simulink model "v1bate3"  (Simulink 8.8)
settings: Solver=ode3  StartTime=0.0  StopTime=inf  FixedStep=0.001  RelTol=1e-3  EnableMultiTasking=on
undefined symbols (not defined in the file): mdaadlink6208
libraries: simulink x19
(part 2 of 2)

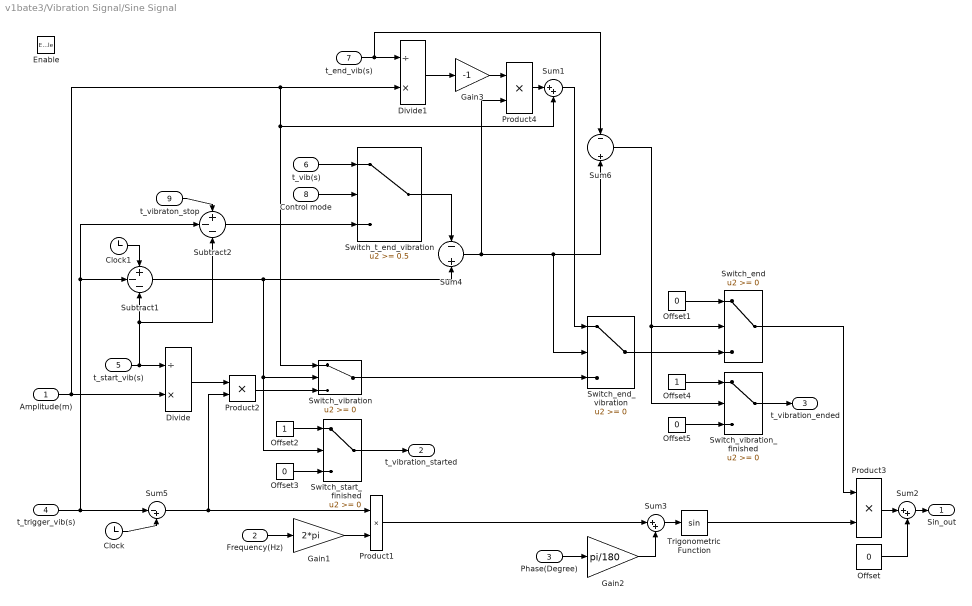
== system v1bate3/Vibration Signal/Sine Signal ==
  Amplitude(m) : Inport
  Frequency(Hz) : Inport  Port=2
  Phase(Degree) : Inport  Port=3
  t_trigger_vib(s) : Inport  Port=4
  t_start_vib(s) : Inport  Port=5
  t_vib(s) : Inport  Port=6
  t_end_vib(s) : Inport  Port=7
  Control mode : Inport  Port=8
  t_vibraton_stop : Inport  Port=9
  Enable : EnablePort  StatesWhenEnabling=reset
  Clock : Clock
      settings: Decimation=100
  Clock1 : Clock
      settings: Decimation=100
  Divide : Product  Inputs=/*
  Divide1 : Product  Inputs=/*
  Gain1 : Gain  Gain=2*pi  SaturateOnIntegerOverflow=on  OutDataTypeStr=Inherit: Same as input  ParamDataTypeStr=Inherit: Same as input
  Gain2 : Gain  Gain=pi/180  SaturateOnIntegerOverflow=on  OutDataTypeStr=Inherit: Same as input  ParamDataTypeStr=Inherit: Same as input
  Gain3 : Gain  Gain=-1  SaturateOnIntegerOverflow=on  OutDataTypeStr=Inherit: Same as input  ParamDataTypeStr=Inherit: Same as input
  Offset{,1,3,5} (4 alike) : Constant  Value=0
  Offset2 : Constant
  Offset4 : Constant
  Product1 : Product  SaturateOnIntegerOverflow=on  OutDataTypeStr=Inherit: Same as first input
  Product2 : Product  RndMeth=Zero
  Product3 : Product  SaturateOnIntegerOverflow=on  OutDataTypeStr=Inherit: Same as first input
  Product4 : Product  RndMeth=Zero
  Subtract1 : Sum  Inputs=+--
  Subtract2 : Sum  Inputs=+--
  Sum1 : Sum  Inputs=|++  SaturateOnIntegerOverflow=on
  Sum2 : Sum  Inputs=|++  SaturateOnIntegerOverflow=on
  Sum3 : Sum  Inputs=|++  SaturateOnIntegerOverflow=on
  Sum4 : Sum  Inputs=-+  SaturateOnIntegerOverflow=on
  Sum5 : Sum  Inputs=|-+  SaturateOnIntegerOverflow=on
  Sum6 : Sum  Inputs=-||+  SaturateOnIntegerOverflow=on
  Switch_end : Switch
  Switch_end_vibration : Switch
  Switch_start_finished : Switch
  Switch_t_end_vibration : Switch  Threshold=0.5
  Switch_vibration : Switch
  Switch_vibration_finished : Switch
  Trigonometric Function : Trigonometry
  Sin_out : Outport
  t_vibration_started : Outport  Port=2
  t_vibration_ended : Outport  Port=3
  wires:
  Product3/1 -> Sum2/1
  Sum2/1 -> Sin_out/1
  Offset/1 -> Sum2/2
  Frequency(Hz)/1 -> Gain1/1
  Sum3/1 -> Trigonometric Function/1
  Trigonometric Function/1 -> Product3/2
  Product1/1 -> Sum3/1
  Gain2/1 -> Sum3/2
  Phase(Degree)/1 -> Gain2/1
  t_trigger_vib(s)/1 -> Sum5/1, Subtract2/2, Subtract1/2
  Sum5/1 -> Product1/1, Product2/2
  Gain1/1 -> Product1/2
  Clock1/1 -> Subtract1/1
  Subtract1/1 -> Sum4/2, Switch_start_finished/2, Switch_vibration/2
  Product2/1 -> Switch_vibration/3
  Switch_vibration/1 -> Switch_end_vibration/3
  Switch_end_vibration/1 -> Switch_end/3
  Switch_end/1 -> Product3/1
  Sum6/1 -> Switch_vibration_finished/2, Switch_end/2
  Divide1/1 -> Gain3/1
  Gain3/1 -> Product4/1
  Offset1/1 -> Switch_end/1
  Sum4/1 -> Product4/2, Switch_end_vibration/2, Sum6/2
  t_end_vib(s)/1 -> Divide1/1, Sum6/1
  Product4/1 -> Sum1/1
  Divide/1 -> Product2/1
  t_start_vib(s)/1 -> Divide/1, Subtract1/3, Subtract2/3
  Amplitude(m)/1 -> Divide/2, Divide1/2, Switch_vibration/1, Sum1/2
  Sum1/1 -> Switch_end_vibration/1
  Switch_start_finished/1 -> t_vibration_started/1
  Offset2/1 -> Switch_start_finished/1
  Offset3/1 -> Switch_start_finished/3
  Switch_vibration_finished/1 -> t_vibration_ended/1
  Offset4/1 -> Switch_vibration_finished/1
  Offset5/1 -> Switch_vibration_finished/3
  Clock/1 -> Sum5/2
  Control mode/1 -> Switch_t_end_vibration/2
  t_vib(s)/1 -> Switch_t_end_vibration/1
  t_vibraton_stop/1 -> Subtract2/1
  Subtract2/1 -> Switch_t_end_vibration/3
  Switch_t_end_vibration/1 -> Sum4/1

== system v1bate3/Vibration Signal/Vibration start trigger ==
  In1 : Inport
  Trigger : TriggerPort  VariantControl=Variant
  Out1 : Outport
  wires:
  In1/1 -> Out1/1

== system v1bate3/Vibration Signal/Vibration stop trigger ==
  In1 : Inport
  Trigger : TriggerPort  VariantControl=Variant
  Out1 : Outport
  wires:
  In1/1 -> Out1/1

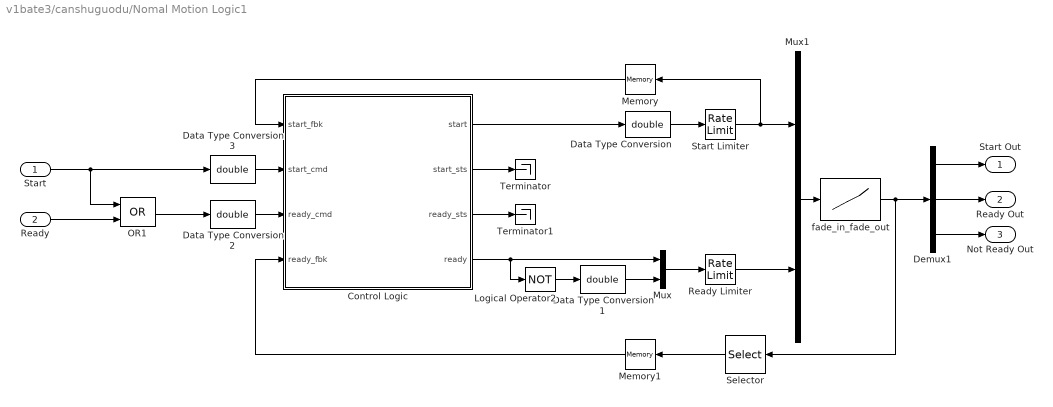
== system v1bate3/canshuguodu/Nomal Motion Logic1 ==
  Start : Inport
  Ready : Inport  Port=2
  Control Logic : Stateflow chart  TreatAsAtomicUnit=on
  Data Type Conversion{,1..3} (4 alike) : DataTypeConversion  OutDataTypeStr=double  SaturateOnIntegerOverflow=on  RndMeth=Zero
  Demux1 : Demux  Outputs=3
  Logical Operator2 : Logic  Operator=NOT  Inputs=3  AllPortsSameDT=off
  Memory : Memory
  Memory1 : Memory
  Mux : Mux  Inputs=2
  Mux1 : Mux  Inputs=2
  OR1 : Logic  Operator=OR  AllPortsSameDT=off
  Ready Limiter : RateLimiter  RisingSlewLimit=1/20  FallingSlewLimit=-1/20
  Selector : Selector  InputPortWidth=3  IndexOptions=Index vector (dialog)  Indices=[2]  OutputSizes=1
  Start Limiter : RateLimiter  RisingSlewLimit=1/3  FallingSlewLimit=-1/3
  Terminator : Terminator
  Terminator1 : Terminator
  fade_in_fade_out : Lookup  InputValues=[0:0.001:1]  Table=(sin(([0:0.001:1]*2-1)*pi/2)+1)/2  SaturateOnIntegerOverflow=on
  Start Out : Outport
  Ready Out : Outport  Port=2
  Not Ready Out : Outport  Port=3
  wires:
  Ready/1 -> OR1/2
  Start/1 -> OR1/1, Data Type Conversion3/1
  Control Logic/3(ready_sts) -> Terminator1/1
  Control Logic/2(start_sts) -> Terminator/1
  OR1/1 -> Data Type Conversion2/1
  Data Type Conversion3/1 -> Control Logic/2(start_cmd)
  Demux1/3 -> Not Ready Out/1
  Demux1/1 -> Start Out/1
  Demux1/2 -> Ready Out/1
  Data Type Conversion/1 -> Start Limiter/1
  Start Limiter/1 -> Mux1/1, Memory/1
  Control Logic/1(start) -> Data Type Conversion/1
  Control Logic/4(ready) -> Logical Operator2/1, Mux/1
  Logical Operator2/1 -> Data Type Conversion1/1
  Mux/1 -> Ready Limiter/1
  Ready Limiter/1 -> Mux1/2
  Mux1/1 -> fade_in_fade_out/1
  fade_in_fade_out/1 -> Selector/1, Demux1/1
  Memory/1 -> Control Logic/1(start_fbk)
  Memory1/1 -> Control Logic/4(ready_fbk)
  Data Type Conversion1/1 -> Mux/2
  Data Type Conversion2/1 -> Control Logic/3(ready_cmd)
  Selector/1 -> Memory1/1

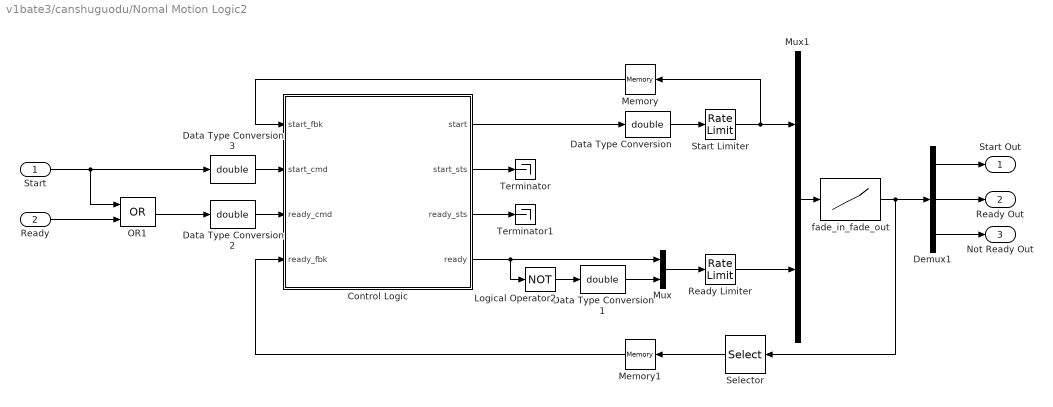
== system v1bate3/canshuguodu/Nomal Motion Logic2 ==
  Start : Inport
  Ready : Inport  Port=2
  Control Logic : Stateflow chart  TreatAsAtomicUnit=on
  Data Type Conversion{,1..3} (4 alike) : DataTypeConversion  OutDataTypeStr=double  SaturateOnIntegerOverflow=on  RndMeth=Zero
  Demux1 : Demux  Outputs=3
  Logical Operator2 : Logic  Operator=NOT  Inputs=3  AllPortsSameDT=off
  Memory : Memory
  Memory1 : Memory
  Mux : Mux  Inputs=2
  Mux1 : Mux  Inputs=2
  OR1 : Logic  Operator=OR  AllPortsSameDT=off
  Ready Limiter : RateLimiter  RisingSlewLimit=1/20  FallingSlewLimit=-1/20
  Selector : Selector  InputPortWidth=3  IndexOptions=Index vector (dialog)  Indices=[2]  OutputSizes=1
  Start Limiter : RateLimiter  RisingSlewLimit=1/3  FallingSlewLimit=-1/3
  Terminator : Terminator
  Terminator1 : Terminator
  fade_in_fade_out : Lookup  InputValues=[0:0.001:1]  Table=(sin(([0:0.001:1]*2-1)*pi/2)+1)/2  SaturateOnIntegerOverflow=on
  Start Out : Outport
  Ready Out : Outport  Port=2
  Not Ready Out : Outport  Port=3
  wires:
  Ready/1 -> OR1/2
  Start/1 -> OR1/1, Data Type Conversion3/1
  Control Logic/3(ready_sts) -> Terminator1/1
  Control Logic/2(start_sts) -> Terminator/1
  OR1/1 -> Data Type Conversion2/1
  Data Type Conversion3/1 -> Control Logic/2(start_cmd)
  Demux1/3 -> Not Ready Out/1
  Demux1/1 -> Start Out/1
  Demux1/2 -> Ready Out/1
  Data Type Conversion/1 -> Start Limiter/1
  Start Limiter/1 -> Mux1/1, Memory/1
  Control Logic/1(start) -> Data Type Conversion/1
  Control Logic/4(ready) -> Logical Operator2/1, Mux/1
  Logical Operator2/1 -> Data Type Conversion1/1
  Mux/1 -> Ready Limiter/1
  Ready Limiter/1 -> Mux1/2
  Mux1/1 -> fade_in_fade_out/1
  fade_in_fade_out/1 -> Selector/1, Demux1/1
  Memory/1 -> Control Logic/1(start_fbk)
  Memory1/1 -> Control Logic/4(ready_fbk)
  Data Type Conversion1/1 -> Mux/2
  Data Type Conversion2/1 -> Control Logic/3(ready_cmd)
  Selector/1 -> Memory1/1

== system v1bate3/huituixinhao1/Triggered Subsystem2 ==
  Trigger : TriggerPort  VariantControl=Variant
  Digital Clock : DigitalClock  SampleTime=-1
  force-single1 : Outport
  wires:
  Digital Clock/1 -> force-single1/1

== system v1bate3/jiechuhuitui2/Triggered Subsystem1 ==
  Trigger : TriggerPort  VariantControl=Variant
  c3 : Constant
  force-single1 : Outport
  wires:
  c3/1 -> force-single1/1

== system v1bate3/jiechuhuitui2/Triggered Subsystem2 ==
  Trigger : TriggerPort  TriggerType=falling  VariantControl=Variant
  c3 : Constant
  force-single1 : Outport
  wires:
  c3/1 -> force-single1/1

== system v1bate3/single with d/Triggered Subsystem1 ==
  Trigger : TriggerPort  VariantControl=Variant
  c7 : Constant
  tingzhenxinhao : Outport
  wires:
  c7/1 -> tingzhenxinhao/1

== system v1bate3/single with d/Triggered Subsystem2 ==
  Trigger : TriggerPort  VariantControl=Variant
  Digital Clock : DigitalClock  SampleTime=-1
  force-single1 : Outport
  wires:
  Digital Clock/1 -> force-single1/1

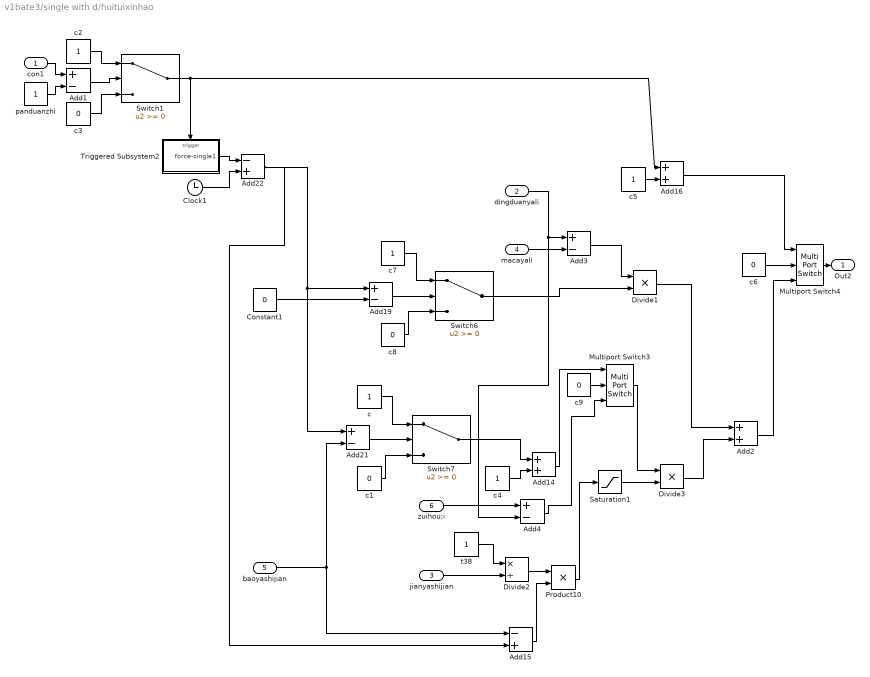
== system v1bate3/single with d/huituixinhao ==
  con1 : Inport
  dingduanyali : Inport  Port=2
  jianyashijian : Inport  Port=3
  macayali : Inport  Port=4
  baoyashijian : Inport  Port=5
  zuihou;i : Inport  Port=6
  Add{1,3..4,19,21} (5 alike) : Sum  Inputs=+-
  Add14 : Sum
  Add15 : Sum  Inputs=-+
  Add16 : Sum
  Add2 : Sum
  Add22 : Sum  Inputs=-+
  Clock1 : Clock
  Constant1 : Constant  Value=0
  Divide1 : Product  Inputs=**
  Divide2 : Product  Inputs=*/
  Divide3 : Product  Inputs=**
  Multiport Switch3 : MultiPortSwitch  Inputs=2
  Multiport Switch4 : MultiPortSwitch  Inputs=2
  Product10 : Product  RndMeth=Zero
  Saturation1 : Saturate  UpperLimit=1  LowerLimit=-1
  Switch1 : Switch
  Switch6 : Switch
  Switch7 : Switch
  Triggered Subsystem2 : Subsystem  TreatAsAtomicUnit=on
  c{,2,4..5,7} (5 alike) : Constant
  c{1,3,6,8..9} (5 alike) : Constant  Value=0
  panduanzhi : Constant
  t38 : Constant
  Out2 : Outport
  wires:
  Triggered Subsystem2/1(force-single1) -> Add22/1
  Clock1/1 -> Add22/2
  t38/1 -> Divide2/1
  Product10/1 -> Saturation1/1
  Saturation1/1 -> Divide3/2
  Divide2/1 -> Product10/1
  Add15/1 -> Product10/2
  baoyashijian/1 -> Add15/1, Add21/2
  Multiport Switch3/1 -> Divide3/1
  c/1 -> Switch7/1
  c1/1 -> Switch7/3
  Add21/1 -> Switch7/2
  c9/1 -> Multiport Switch3/2
  Add14/1 -> Multiport Switch3/1
  Switch7/1 -> Add14/1
  c4/1 -> Add14/2
  Add22/1 -> Add15/2, Add21/1, Add19/1
  panduanzhi/1 -> Add1/2
  Add1/1 -> Switch1/2
  c2/1 -> Switch1/1
  c3/1 -> Switch1/3
  Switch1/1 -> Triggered Subsystem2/Trigger, Add16/1
  Add4/1 -> Multiport Switch3/3
  con1/1 -> Add1/1
  jianyashijian/1 -> Divide2/2
  c6/1 -> Multiport Switch4/2
  Add16/1 -> Multiport Switch4/1
  Multiport Switch4/1 -> Out2/1
  c5/1 -> Add16/2
  Divide3/1 -> Add2/2
  Add2/1 -> Multiport Switch4/3
  c7/1 -> Switch6/1
  c8/1 -> Switch6/3
  Add19/1 -> Switch6/2
  Constant1/1 -> Add19/2
  dingduanyali/1 -> Add3/1, Add4/2
  macayali/1 -> Add3/2
  Add3/1 -> Divide1/1
  Switch6/1 -> Divide1/2
  Divide1/1 -> Add2/1
  zuihou;i/1 -> Add4/1

== system v1bate3/single with time1/Triggered Subsystem2 ==
  Trigger : TriggerPort  VariantControl=Variant
  Digital Clock : DigitalClock  SampleTime=-1
  force-single1 : Outport
  wires:
  Digital Clock/1 -> force-single1/1

== system v1bate3/tvc_filter1/filter ==
  uxa : Inport
  Dxf : Gain  Gain=0.5*6.28*0.5*6.28  SaturateOnIntegerOverflow=on  OutDataTypeStr=Inherit: Same as input  ParamDataTypeStr=Inherit: Same as input
  Integrator : Integrator
  Integrator1 : Integrator
  Sum : Sum  Inputs=+--  SaturateOnIntegerOverflow=on
  Vxf : Gain  Gain=2*0.7*0.5*6.28  SaturateOnIntegerOverflow=on  OutDataTypeStr=Inherit: Same as input  ParamDataTypeStr=Inherit: Same as input
  ax : Outport
  vx : Outport  Port=2
  dx : Outport  Port=3
  wires:
  Integrator1/1 -> Dxf/1, dx/1
  uxa/1 -> Sum/1
  Dxf/1 -> Sum/2
  Vxf/1 -> Sum/3
  Integrator/1 -> vx/1, Vxf/1, Integrator1/1
  Sum/1 -> ax/1, Integrator/1

== system v1bate3/single with d/huituixinhao/Triggered Subsystem2 ==
  Trigger : TriggerPort  VariantControl=Variant
  Digital Clock : DigitalClock  SampleTime=-1
  force-single1 : Outport
  wires:
  Digital Clock/1 -> force-single1/1

== stateflow chart canshuguodu/Nomal Motion Logic1/Control Logic ==
  state run_mode [parallel]
    settings: executionOrder=1
    state running
      du:start=1;start_sts=2;
    state to_stopped
      du:start=0;start_sts=3;
    state to_running
      du:start=1;start_sts=1;
    state stopped
      du:start=0;start_sts=0;
    to_running -> running [order 1] : [start_cmd==start_fbk]
    running -> to_stopped : [!start_cmd]
    to_stopped -> to_running [order 1] : [start_cmd&&in(ready_mode.ready)]
    to_running -> to_stopped [order 2] : [!start_cmd]
    to_stopped -> stopped [order 2] : [start_cmd==start_fbk]
    stopped -> to_running : [start_cmd&&in(ready_mode.ready)]
    (default) -> stopped
  state ready_mode [parallel]
    settings: executionOrder=2
    state ready
      du:ready=1;ready_sts=2;
    state to_rest
      du:ready=0;ready_sts=3;
    state rest
      du:ready=0;ready_sts=0;
    state to_ready
      du:ready=1;ready_sts=1;
    ready -> to_rest : [!ready_cmd&&in(run_mode.stopped)]
    to_ready -> ready [order 1] : [ready_cmd==ready_fbk]
    to_rest -> to_ready [order 1] : [ready_cmd]
    to_ready -> to_rest [order 2] : [!ready_cmd&&in(run_mode.stopped)]
    to_rest -> rest [order 2] : [ready_cmd==ready_fbk]
    rest -> to_ready : [ready_cmd]
    (default) -> rest
  data: start_fbk input double; start_cmd input double; ready_cmd input double; ready_fbk input double; start output boolean; start_sts output double; ready_sts output double; ready output boolean

== stateflow chart canshuguodu/Nomal Motion Logic2/Control Logic ==
  state run_mode [parallel]
    settings: executionOrder=1
    state running
      du:start=1;start_sts=2;
    state to_stopped
      du:start=0;start_sts=3;
    state to_running
      du:start=1;start_sts=1;
    state stopped
      du:start=0;start_sts=0;
    to_running -> running [order 1] : [start_cmd==start_fbk]
    running -> to_stopped : [!start_cmd]
    to_stopped -> to_running [order 1] : [start_cmd&&in(ready_mode.ready)]
    to_running -> to_stopped [order 2] : [!start_cmd]
    to_stopped -> stopped [order 2] : [start_cmd==start_fbk]
    stopped -> to_running : [start_cmd&&in(ready_mode.ready)]
    (default) -> stopped
  state ready_mode [parallel]
    settings: executionOrder=2
    state ready
      du:ready=1;ready_sts=2;
    state to_rest
      du:ready=0;ready_sts=3;
    state rest
      du:ready=0;ready_sts=0;
    state to_ready
      du:ready=1;ready_sts=1;
    ready -> to_rest : [!ready_cmd&&in(run_mode.stopped)]
    to_ready -> ready [order 1] : [ready_cmd==ready_fbk]
    to_rest -> to_ready [order 1] : [ready_cmd]
    to_ready -> to_rest [order 2] : [!ready_cmd&&in(run_mode.stopped)]
    to_rest -> rest [order 2] : [ready_cmd==ready_fbk]
    rest -> to_ready : [ready_cmd]
    (default) -> rest
  data: start_fbk input double; start_cmd input double; ready_cmd input double; ready_fbk input double; start output boolean; start_sts output double; ready_sts output double; ready output boolean

== stateflow chart Nomal Motion Logic/Control Logic ==
  state run_mode [parallel]
    settings: executionOrder=1
    state running
      du:start=1;start_sts=2;
    state to_stopped
      du:start=0;start_sts=3;
    state to_running
      du:start=1;start_sts=1;
    state stopped
      du:start=0;start_sts=0;
    to_running -> running [order 1] : [start_cmd==start_fbk]
    running -> to_stopped : [!start_cmd]
    to_stopped -> to_running [order 1] : [start_cmd&&in(ready_mode.ready)]
    to_running -> to_stopped [order 2] : [!start_cmd]
    stopped -> to_running : [start_cmd&&in(ready_mode.ready)]
    to_stopped -> stopped [order 2] : [start_cmd==start_fbk]
    (default) -> stopped
  state ready_mode [parallel]
    settings: executionOrder=2
    state ready
      du:ready=1;ready_sts=2;
    state to_rest
      du:ready=0;ready_sts=3;
    state rest
      du:ready=0;ready_sts=0;
    state to_ready
      du:ready=1;ready_sts=1;
    to_ready -> ready [order 1] : [ready_cmd==ready_fbk]
    ready -> to_rest : [!ready_cmd&&in(run_mode.stopped)]
    to_rest -> to_ready [order 1] : [ready_cmd]
    to_ready -> to_rest [order 2] : [!ready_cmd&&in(run_mode.stopped)]
    rest -> to_ready : [ready_cmd]
    to_rest -> rest [order 2] : [ready_cmd==ready_fbk]
    (default) -> rest
  data: start_fbk input double; start_cmd input double; ready_cmd input double; ready_fbk input double; start output boolean; start_sts output double; ready_sts output double; ready output boolean
